simulink model "fixedVsVariable"  (R2018a)
settings: Solver=VariableStepDiscrete  StartTime=0.0  StopTime=20.0  RelTol=1e-3
settings Model: Creator=gchandra  LastModifiedBy=bneiswan
settings DataIOCC: LimitDataPoints=on  SaveFormat=Array  SignalLoggingName=sigsOut
settings OptimizationCC: ExpressionDepthLimit=2147483647  InitFltsAndDblsToZero=on  LifeSpan=inf
settings DebuggingCC: SaveWithParameterizedLinksMsg=none  UnderspecifiedInitializationDetection=Classic  MergeDetectMultiDrivingBlocksExec=none  SignalResolutionControl=TryResolveAllWithWarning  MultiTaskDSMMsg=warning  MultiTaskCondExecSysMsg=none  ParameterPrecisionLossMsg=none  FcnCallInpInsideContextMsg=warning  AllowSymbolicDim=off  StateNameClashWarn=warning  SFUnexpectedBacktrackingDiag=warning  SFNoUnconditionalDefaultTransitionDiag=warning  SFExecutionAtInitializationDiag=none
settings HardwareCC: ProdBitPerPointer=32  ProdBitPerSizeT=32  ProdBitPerPtrDiffT=32  ProdLargestAtomicFloat=None  ProdIntDivRoundTo=Undefined  ProdEndianess=Unspecified  ProdWordSize=32  ProdHWDeviceType=32-bit Generic  TargetUnknown=on
settings ModelReferenceCC: PropagateSignalLabelsOutOfModel=off
settings CodeAppCC: StateflowObjectComments=on
settings GRTTargetCC: TargetFcnLib=ansi_tfl_tmw.mat  TargetLangStandard=C89/C90 (ANSI)  GeneratePreprocessorConditionals=Disable all  CombineOutputUpdateFcns=off  GRTInterface=on
settings ConfigComp: CovMetricSettings=dw  CovHtmlReporting=on  CovSaveCumulativeToWorkspaceVar=on  CovSaveSingleToWorkspaceVar=on  CovExternalEMLEnable=off  CovSFcnEnable=off

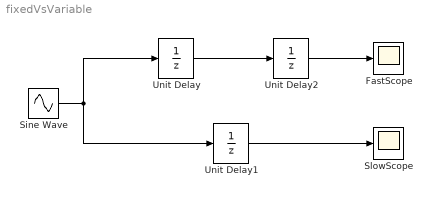
== system fixedVsVariable ==
  FastScope : Scope
  Sine Wave : Sin  SampleTime=0
  SlowScope : Scope
  Unit Delay : UnitDelay  SampleTime=0.4
      settings: AttributesFormatString=Sampling Time: %<SampleTime>
  Unit Delay1 : UnitDelay  SampleTime=.6
      settings: AttributesFormatString=Sampling Time: %<SampleTime>
  Unit Delay2 : UnitDelay  SampleTime=0.4
      settings: AttributesFormatString=Sampling Time: %<SampleTime>
  wires:
  Sine Wave/1 -> Unit Delay/1, Unit Delay1/1
  Unit Delay/1 -> Unit Delay2/1
  Unit Delay2/1 -> FastScope/1
  Unit Delay1/1 -> SlowScope/1
